simulink model "sim1"  (R2018a)
settings: Solver=VariableStepAuto  StartTime=0.0  StopTime=5  RelTol=1e-3
libraries: simulink x2
settings Model: Creator=Dell  LastModifiedBy=Dell

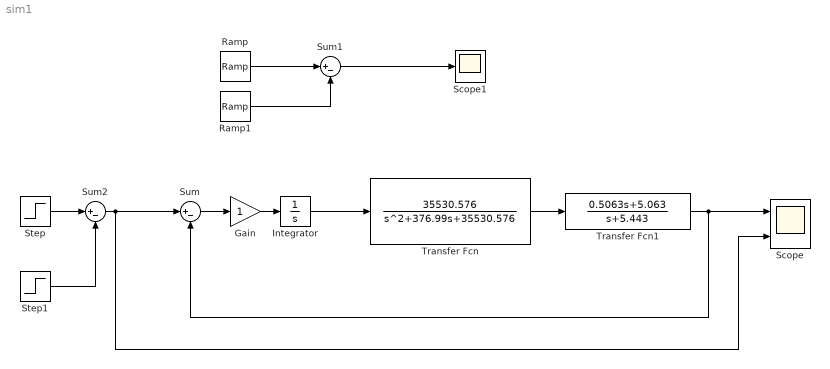
== system sim1 ==
  Gain : Gain
  Integrator : Integrator
  Ramp : simulink/Sources/Ramp  slope=150  start=1  InitialOutput=5
  Ramp1 : simulink/Sources/Ramp  slope=150  start=1.1  InitialOutput=0
  Scope : Scope  NumInputPorts=2
  Scope1 : Scope
  Step : Step  Before=5  After=20  SampleTime=0
  Step1 : Step  Time=5  After=15  SampleTime=0
  Sum : Sum  Inputs=|+-
  Sum1 : Sum  Inputs=|+-
  Sum2 : Sum  Inputs=|+-
  Transfer Fcn : TransferFcn  Numerator=[35530.576]  Denominator=[1 376.99 35530.576]
  Transfer Fcn1 : TransferFcn  Numerator=[0.5063 5.063]  Denominator=[1 5.443]
  wires:
  Gain/1 -> Integrator/1
  Sum/1 -> Gain/1
  Transfer Fcn/1 -> Transfer Fcn1/1
  Integrator/1 -> Transfer Fcn/1
  Sum2/1 -> Scope/2, Sum/1
  Transfer Fcn1/1 -> Scope/1, Sum/2
  Step/1 -> Sum2/1
  Step1/1 -> Sum2/2
  Ramp/1 -> Sum1/1
  Ramp1/1 -> Sum1/2
  Sum1/1 -> Scope1/1
